simulink model "GA_LQR_sim"  (R2023a)
settings: Solver=VariableStepAuto  StartTime=0.0  StopTime=10  FixedStep=1e-3  RelTol=1e-3
InitFcn:
  | m0=0.8; m1=0.5; m2=0.3; L1=0.3; L2=0.2; l1=0.15; l2=0.1; I1=0.015; I2=0.004; g=9.8;
  | d1=(m0+m1+m2);
  | d2=(m1*l1+m2*L1);
  | d3=m1*l1^2+m2*L1^2+I1;
  | d4=m2*l2;
  | d5=m2*L1*l2;
  | d6=m2*l2^2+I2;
settings Model: Creator=luand  LastModifiedBy=luand
settings DataIOCC: ReturnWorkspaceOutputs=off

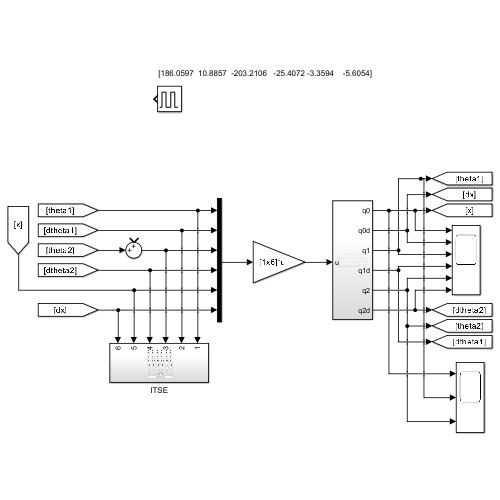
[thumbnail: Simulink's stored preview of the top-level diagram]
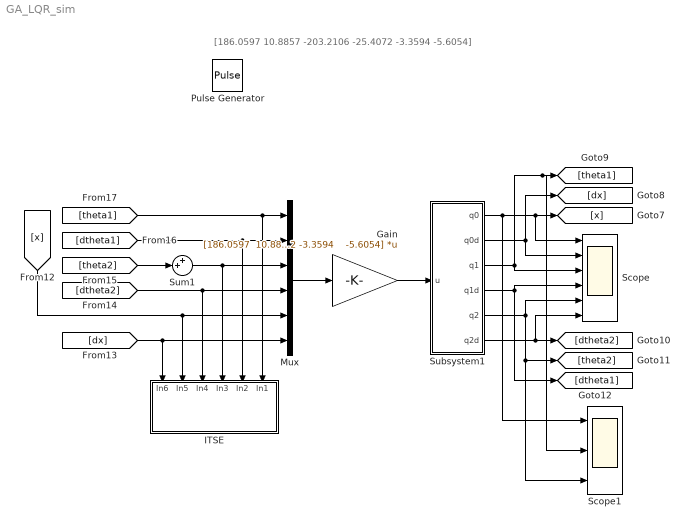
== system GA_LQR_sim ==
  note: [186.0597 10.8857 -203.2106 -25.4072 -3.3594 -5.6054]
  Gain : Gain  Gain="[186.0597  10.8857  -203.2106   -25.4072 -3.3594    -5.6054]"  Multiplication=Matrix(K*u)
  ITSE : Subsystem
      settings: PortSchema="{\"entries\":[{\"content\":{\"sides\":[{\"content\":{},\"type\":\"ConnectorPlacement.EquallySpacedRectSide\",\"uuid\":\"e58fb5c4-5c40-438f-82d2-64df3ffab965\"},{\"content\":{\"side\":\"RIGHT\"},\"type\":\"ConnectorPlacement.EquallySpacedRectSide\",\"uuid\":\"eaea93d5-b103-43eb-bbad-e2254ba1d517\"},{\"content\":{\"connectorIds\":[\"In1\",\"In2\",\"In3\",\"In4\",\"In5\",\"In6\"],\"side\":\"TOP\"},\"type\":\"ConnectorPlacement.EquallySpacedRectSide\",\"uuid\":\"3ee734ab-a155-4509-a0f5-708cc4a4cdab\"}]},\"type\":\"ConnectorPlacement.EquallySpacedConnector\",\"uuid\":\"a98ea38b-27a9-4338-8328-bf891ae89dad\"}],\"packageUris\":[\"http://schema.mathworks.com/mf0/Connector/R2020b\"],\"version\":\"1.0\"}"
  Mux : Mux  Inputs=6
  Pulse Generator : DiscretePulseGenerator  PulseType=Time based  Amplitude=pi/80  Period=5  PulseWidth=10
  Scope : Scope  NumInputPorts=6
  Scope1 : Scope  NumInputPorts=3
  Subsystem1 : Subsystem
  Sum1 : Sum  Inputs=++|
  wires:
  Subsystem1/1(q0) -> Scope1/1, Scope/1, [x]
  [x] -> ITSE/5(In5), Mux/5
  Subsystem1/3(q1) -> Scope/3, [theta1], Scope1/2
  Subsystem1/5(q2) -> Scope/5, [theta2], Scope1/3
  Subsystem1/2(q0d) -> Scope/2, [dx]
  Subsystem1/6(q2d) -> [dtheta2], Scope/6
  Subsystem1/4(q1d) -> Scope/4, [dtheta1]
  Mux/1 -> Gain/1
  [dx] -> Mux/6, ITSE/6(In6)
  [dtheta2] -> Mux/4, ITSE/4(In4)
  [dtheta1] -> Mux/2, ITSE/2(In2)
  [theta1] -> Mux/1, ITSE/1(In1)
  Gain/1 -> Subsystem1/1(u)
  Sum1/1 -> ITSE/3(In3), Mux/3
  [theta2] -> Sum1/2

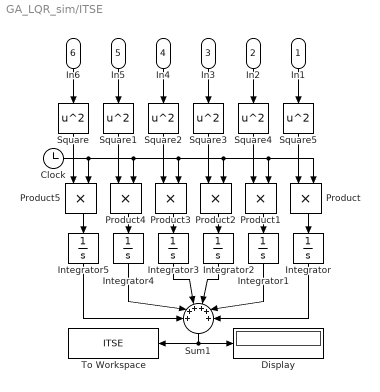
== system GA_LQR_sim/ITSE ==
  In1 : Inport
  In2 : Inport  Port=2
  In3 : Inport  Port=3
  In4 : Inport  Port=4
  In5 : Inport  Port=5
  In6 : Inport  Port=6
  Clock : Clock
  Display : Display
  Integrator{,1..5} (6 alike) : Integrator
  Product{,1..5} (6 alike) : Product
  Square{,1..5} (6 alike) : Math  Operator=square
  Sum1 : Sum  Inputs=++++++
  To Workspace : ToWorkspace  VariableName=ITSE  SampleTime=-1
  wires:
  Clock/1 -> Product/2, Product1/2, Product2/2, Product3/2, Product4/2, Product5/2
  Product3/1 -> Integrator3/1
  Square5/1 -> Product/1
  Integrator/1 -> Sum1/6
  In4/1 -> Square2/1
  Integrator4/1 -> Sum1/2
  Product/1 -> Integrator/1
  Product2/1 -> Integrator2/1
  Integrator3/1 -> Sum1/3
  Integrator2/1 -> Sum1/4
  Integrator1/1 -> Sum1/5
  Product4/1 -> Integrator4/1
  Sum1/1 -> Display/1, To Workspace/1
  Integrator5/1 -> Sum1/1
  Square/1 -> Product5/1
  Product5/1 -> Integrator5/1
  Square4/1 -> Product1/1
  Square3/1 -> Product2/1
  In2/1 -> Square4/1
  Product1/1 -> Integrator1/1
  Square1/1 -> Product4/1
  Square2/1 -> Product3/1
  In5/1 -> Square1/1
  In6/1 -> Square/1
  In3/1 -> Square3/1
  In1/1 -> Square5/1

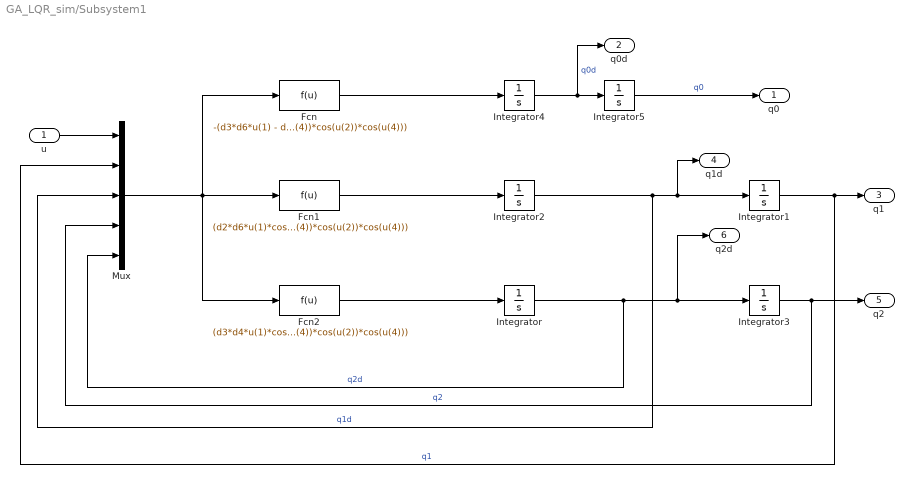
== system GA_LQR_sim/Subsystem1 ==
  u : Inport
  Fcn : Fcn  Expr=-(d3*d6*u(1) - d5^2*u(1)*cos(u(2) - u(4))^2 + d2*d3*d6*u(3)^2*sin(u(2)) + d3*d4*d6*u(5)^2*sin(u(4)) - d2*d5^2*u(3)^2*cos(u(2) - u(4))^2*sin(u(2)) - d4*d5^2*u(5)^2*cos(u(2) - u(4))^2*sin(u(4)) - d2^2*d6*g*cos(u(2))*sin(u(2)) - d3*d4^2*g*cos(u(4))*sin(u(4)) + d2*d5^2*u(3)^2*cos(u(2) - u(4))*sin(u(2) - u(4))*cos(u(2)) - d4*d5^2*u(5)^2*cos(u(2) - u(4))*sin(u(2) - u(4))*cos(u(4)) - d3*d4*d5*u(3)^2*sin(u(2) - u(4))*cos(u(4)) + d2*d5*d6*u(5)^2*sin(u(2) - u(4))*cos(u(2)) + d2*d4*d5*g*cos(u(2) - u(4))*cos(u(2))*sin(u(4)) + d2*d4*d5*g*cos(u(2) - u(4))*cos(u(4))*sin(u(2)))/(d3*d4^2*cos(u(4))^2 - d1*d3*d6 + d2^2*d6*cos(u(2))^2 + d1*d5^2*cos(u(2) - u(4))^2 - 2*d2*d4*d5*cos(u(2) - u(4))*cos(u(2))*cos(u(4)))
  Fcn1 : Fcn  Expr=(d2*d6*u(1)*cos(u(2)) + d2*d4^2*g*cos(u(4))^2*sin(u(2)) + d2^2*d6*u(3)^2*cos(u(2))*sin(u(2)) + d1*d5^2*u(3)^2*cos(u(2) - u(4))*sin(u(2) - u(4)) + d1*d5*d6*u(5)^2*sin(u(2) - u(4)) - d4*d5*u(1)*cos(u(2) - u(4))*cos(u(4)) - d4^2*d5*u(5)^2*sin(u(2) - u(4))*cos(u(4))^2 - d1*d2*d6*g*sin(u(2)) - d4^2*d5*u(5)^2*cos(u(2) - u(4))*cos(u(4))*sin(u(4)) + d2*d4*d6*u(5)^2*cos(u(2))*sin(u(4)) - d2*d4^2*g*cos(u(2))*cos(u(4))*sin(u(4)) + d1*d4*d5*g*cos(u(2) - u(4))*sin(u(4)) - d2*d4*d5*u(3)^2*cos(u(2) - u(4))*cos(u(4))*sin(u(2)) - d2*d4*d5*u(3)^2*sin(u(2) - u(4))*cos(u(2))*cos(u(4)))/(d3*d4^2*cos(u(4))^2 - d1*d3*d6 + d2^2*d6*cos(u(2))^2 + d1*d5^2*cos(u(2) - u(4))^2 - 2*d2*d4*d5*cos(u(2) - u(4))*cos(u(2))*cos(u(4)))
  Fcn2 : Fcn  Expr=(d3*d4*u(1)*cos(u(4)) + d2^2*d4*g*cos(u(2))^2*sin(u(4)) + d3*d4^2*u(5)^2*cos(u(4))*sin(u(4)) - d1*d5^2*u(5)^2*cos(u(2) - u(4))*sin(u(2) - u(4)) - d1*d3*d5*u(3)^2*sin(u(2) - u(4)) - d2*d5*u(1)*cos(u(2) - u(4))*cos(u(2)) + d2^2*d5*u(3)^2*sin(u(2) - u(4))*cos(u(2))^2 - d1*d3*d4*g*sin(u(4)) - d2^2*d5*u(3)^2*cos(u(2) - u(4))*cos(u(2))*sin(u(2)) + d2*d3*d4*u(3)^2*cos(u(4))*sin(u(2)) - d2^2*d4*g*cos(u(2))*cos(u(4))*sin(u(2)) + d1*d2*d5*g*cos(u(2) - u(4))*sin(u(2)) - d2*d4*d5*u(5)^2*cos(u(2) - u(4))*cos(u(2))*sin(u(4)) + d2*d4*d5*u(5)^2*sin(u(2) - u(4))*cos(u(2))*cos(u(4)))/(d3*d4^2*cos(u(4))^2 - d1*d3*d6 + d2^2*d6*cos(u(2))^2 + d1*d5^2*cos(u(2) - u(4))^2 - 2*d2*d4*d5*cos(u(2) - u(4))*cos(u(2))*cos(u(4)))
  Integrator : Integrator  LimitOutput=on  UpperSaturationLimit=50  LowerSaturationLimit=-50
  Integrator1 : Integrator  InitialCondition=pi/6  LimitOutput=on  UpperSaturationLimit=10  LowerSaturationLimit=-10
  Integrator2 : Integrator  LimitOutput=on  UpperSaturationLimit=50  LowerSaturationLimit=-50
  Integrator3 : Integrator  InitialCondition=pi/6  LimitOutput=on  UpperSaturationLimit=10  LowerSaturationLimit=-10
  Integrator4 : Integrator  LimitOutput=on  UpperSaturationLimit=10  LowerSaturationLimit=-10
  Integrator5 : Integrator  LimitOutput=on  UpperSaturationLimit=10  LowerSaturationLimit=-10
  Mux : Mux  Inputs=5
  q0 : Outport  VectorParamsAs1DForOutWhenUnconnected=off
  q0d : Outport  Port=2  VectorParamsAs1DForOutWhenUnconnected=off
  q1 : Outport  Port=3  VectorParamsAs1DForOutWhenUnconnected=off
  q1d : Outport  Port=4  VectorParamsAs1DForOutWhenUnconnected=off
  q2 : Outport  Port=5  VectorParamsAs1DForOutWhenUnconnected=off
  q2d : Outport  Port=6  VectorParamsAs1DForOutWhenUnconnected=off
  wires:
  Integrator/1 -> Mux/5, q2d/1, Integrator3/1  "q2d"
  u/1 -> Mux/1
  Integrator1/1 -> Mux/2, q1/1  "q1"
  Integrator4/1 -> q0d/1, Integrator5/1  "q0d"
  Integrator5/1 -> q0/1  "q0"
  Integrator2/1 -> Mux/3, q1d/1, Integrator1/1  "q1d"
  Integrator3/1 -> Mux/4, q2/1  "q2"
  Mux/1 -> Fcn2/1, Fcn/1, Fcn1/1
  Fcn/1 -> Integrator4/1
  Fcn1/1 -> Integrator2/1
  Fcn2/1 -> Integrator/1
